simulink model "Mutriku_TD_V5_Data"  (R2017a)
settings: Solver=ode1  StartTime=Times.Ts  StopTime=Times.Tsim  FixedStep=Times.Ts  RelTol=1e-3  EnableMultiTasking=on
values from neighbouring files (symbols this model uses):
  CL = 1    [Plot_Main_Biradiale.m]
undefined symbols (not defined in the file or in its folder): L, Times, Turb, WaveData, WEC
libraries: simulink x1
settings Model: Creator=FixnBock  LastModifiedBy=Temo
settings SolverCC: AlgebraicLoopSolver=LineSearch
settings DataIOCC: LimitDataPoints=on  SaveFormat=StructureWithTime
settings OptimizationCC: DefaultParameterBehavior=Inlined  LifeSpan=inf
settings DebuggingCC: AlgebraicLoopMsg=error  SFUnexpectedBacktrackingDiag=warning  SFNoUnconditionalDefaultTransitionDiag=warning  SFExecutionAtInitializationDiag=none
settings HardwareCC: ProdBitPerSizeT=32  ProdBitPerPtrDiffT=32  ProdWordSize=32  ProdHWDeviceType=Specified
settings ModelReferenceCC: PropagateSignalLabelsOutOfModel=off
settings RTWCC: TemplateMakefile=RTW.MSVCBuild  Description=Create Visual C/C++ Solution File for Simulink Coder
settings GRTTargetCC: TargetLangStandard=C89/C90 (ANSI)
settings ConfigComp: CovMetricSettings=dw  CovHtmlReporting=on  CovSaveCumulativeToWorkspaceVar=on  CovSaveSingleToWorkspaceVar=on  CovExternalEMLEnable=off

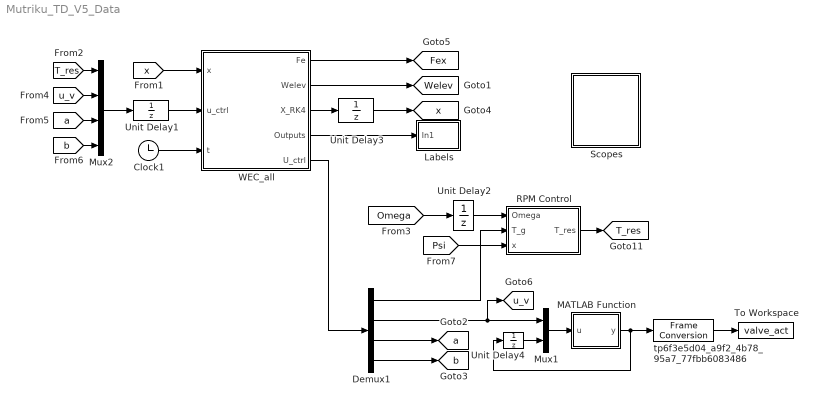
== system Mutriku_TD_V5_Data ==
  Clock1 : Clock
  Demux1 : Demux
  Labels : Subsystem
  MATLAB Function : MATLAB Function  TreatAsAtomicUnit=on
  Mux1 : Mux  Inputs=2
  Mux2 : Mux
  RPM Control : Subsystem
  Scopes : Subsystem
  To Workspace : ToWorkspace  VariableName=valve_act  SampleTime=-1
  Unit Delay1 : UnitDelay  InitialCondition=[0,1,Turb.a,Turb.b]  SampleTime=-1
  Unit Delay2 : UnitDelay  InitialCondition=WEC.Omega0  SampleTime=-1
  Unit Delay3 : UnitDelay  InitialCondition=WEC.X0  SampleTime=-1
  Unit Delay4 : UnitDelay  SampleTime=-1
  WEC_all : MATLAB Function  TreatAsAtomicUnit=on
  tp6f3e5d04_a9f2_4b78_95a7_77fbb6083486 : FrameConversion  InheritSamplingMode=off  OutFrame=Sample-based
  tag scope: Fex=global, T_res=global, Welev=global, a=global, b=global, u_v=global, x=global
  wires:
  tp6f3e5d04_a9f2_4b78_95a7_77fbb6083486/1 -> To Workspace/1
  Unit Delay4/1 -> Mux1/2
  MATLAB Function/1(y) -> Unit Delay4/1, tp6f3e5d04_a9f2_4b78_95a7_77fbb6083486/1
  Mux1/1 -> MATLAB Function/1(u)
  Demux1/2 -> [u_v], Mux1/1
  Demux1/1 -> RPM Control/2(T_g)
  WEC_all/5(U_ctrl) -> Demux1/1
  Clock1/1 -> WEC_all/3(t)
  Unit Delay3/1 -> [x]
  [x] -> WEC_all/1(x)
  WEC_all/4(Outputs) -> Labels/1(In1)
  WEC_all/3(X_RK4) -> Unit Delay3/1
  WEC_all/1(Fe) -> [Fex]
  WEC_all/2(Welev) -> [Welev]
  Demux1/3 -> [a]
  Demux1/4 -> [b]
  [Omega] -> Unit Delay2/1
  Unit Delay2/1 -> RPM Control/1(Omega)
  Mux2/1 -> Unit Delay1/1
  [T_res] -> Mux2/1
  [u_v] -> Mux2/2
  [a] -> Mux2/3
  [b] -> Mux2/4
  Unit Delay1/1 -> WEC_all/2(u_ctrl)
  RPM Control/1(T_res) -> [T_res]
  [Psi] -> RPM Control/3(x)

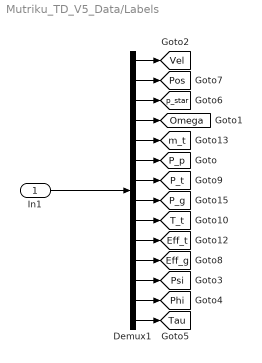
== system Mutriku_TD_V5_Data/Labels ==
  In1 : Inport
  Demux1 : Demux  Outputs=14
  tag scope: Eff_g=global, Eff_t=global, Omega=global, P_g=global, P_p=global, P_t=global, Phi=global, Pos=global, Psi=global, T_t=global, Tau=global, Vel=global, m_t=global, p_star=global
  wires:
  Demux1/5 -> [m_t]
  Demux1/3 -> [p_star]
  Demux1/8 -> [P_g]
  Demux1/1 -> [Vel]
  Demux1/4 -> [Omega]
  Demux1/2 -> [Pos]
  Demux1/9 -> [T_t]
  Demux1/7 -> [P_t]
  Demux1/10 -> [Eff_t]
  Demux1/11 -> [Eff_g]
  Demux1/12 -> [Psi]
  Demux1/13 -> [Phi]
  Demux1/14 -> [Tau]
  Demux1/6 -> [P_p]
  In1/1 -> Demux1/1

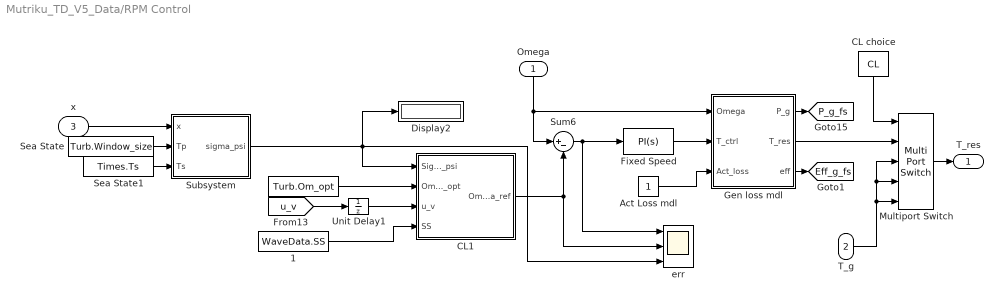
== system Mutriku_TD_V5_Data/RPM Control ==
  Omega : Inport
  T_g : Inport  Port=2
  x : Inport  Port=3
  "    " : Constant  Value=Turb.Om_opt
  "    1" : Constant  Value=WaveData.SS
  Act Loss mdl : Constant
  CL choice : Constant  Value=CL
  CL1 : MATLAB Function  TreatAsAtomicUnit=on
  Display2 : Display
  Fixed Speed : simulink/Continuous/PID Controller  Controller=PI  TimeDomain=Continuous-time  SampleTime=-1  IntegratorMethod=Forward Euler  FilterMethod=Forward Euler  Form=Parallel  UseFilter=on  ControllerParametersSource=internal  P=50  I=0.01  D=0.01  N=100  InitialConditionSource=internal  InitialConditionForIntegrator=0.0  InitialConditionForFilter=0  ExternalReset=none  IgnoreLimit=on  LimitOutput=on  UpperSaturationLimit=Turb.Tmax  LowerSaturationLimit=0  LinearizeAsGain=on  AntiWindupMode=none  Kb=1  TrackingMode=off  Kt=1  PParamMin=[]  PParamMax=[]  IParamMin=[]  IParamMax=[]  DParamMin=[]  DParamMax=[]  NParamMin=[]  NParamMax=[]  KbParamMin=[]  KbParamMax=[]  KtParamMin=[]  KtParamMax=[]  POutMin=[]  POutMax=[]  IOutMin=[]  IOutMax=[]  DOutMin=[]  DOutMax=[]  NOutMin=[]  NOutMax=[]  KbOutMin=[]  KbOutMax=[]  KtOutMin=[]  KtOutMax=[]  IntegratorOutMin=[]  IntegratorOutMax=[]  FilterOutMin=[]  FilterOutMax=[]  SumOutMin=[]  SumOutMax=[]  SumI1OutMin=[]  SumI1OutMax=[]  SumI2OutMin=[]  SumI2OutMax=[]  SumI3OutMin=[]  SumI3OutMax=[]  SumDOutMin=[]  SumDOutMax=[]  SaturationOutMin=[]  SaturationOutMax=[]  IntegratorContinuousStateAttributes=''  IntegratorStateMustResolveToSignalObject=off  IntegratorRTWStateStorageClass=Auto  FilterContinuousStateAttributes=''  FilterStateMustResolveToSignalObject=off  FilterRTWStateStorageClass=Auto  DifferentiatorICPrevScaledInput=0  DifferentiatorOutMin=[]  DifferentiatorOutMax=[]  InitialConditionSetting=State (most efficient)
  Gen loss mdl : MATLAB Function  TreatAsAtomicUnit=on
  Multiport Switch : MultiPortSwitch  Inputs=4  DiagnosticForDefault=None
  Sea State : Constant  Value=Turb.Window_size
  Sea State1 : Constant  Value=Times.Ts
  Subsystem : Subsystem
  Sum6 : Sum  Inputs=|+-
  Unit Delay1 : UnitDelay  InitialCondition=1  SampleTime=-1
  err : Scope  NumInputPorts=3
  T_res : Outport
  tag scope: Eff_g_fs=global, P_g_fs=global
  wires:
  Multiport Switch/1 -> T_res/1
  Omega/1 -> Sum6/1, Gen loss mdl/1(Omega)
  CL choice/1 -> Multiport Switch/1
  CL1/1(Omega_ref) -> Sum6/2, err/2
  T_g/1 -> Multiport Switch/5, Multiport Switch/4, Multiport Switch/3
  Sum6/1 -> Fixed Speed/1, err/1
  Act Loss mdl/1 -> Gen loss mdl/3(Act_loss)
  Gen loss mdl/2(T_res) -> Multiport Switch/2
  Gen loss mdl/1(P_g) -> [P_g_fs]
  Gen loss mdl/3(eff) -> [Eff_g_fs]
  Fixed Speed/1 -> Gen loss mdl/2(T_ctrl)
  "    "/1 -> CL1/2(Omega_opt)
  [u_v] -> Unit Delay1/1
  Unit Delay1/1 -> CL1/3(u_v)
  Sea State/1 -> Subsystem/2(Tp)
  Sea State1/1 -> Subsystem/3(Ts)
  Subsystem/1(sigma_psi) -> err/3, CL1/1(Sigma_psi), Display2/1
  x/1 -> Subsystem/1(x)
  "    1"/1 -> CL1/4(SS)

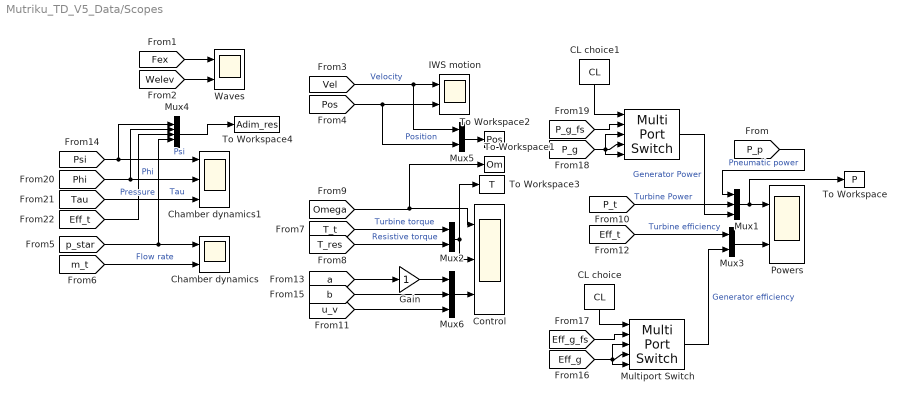
== system Mutriku_TD_V5_Data/Scopes ==
  "    " : MultiPortSwitch  Inputs=4  DiagnosticForDefault=None
  CL choice : Constant  Value=CL
  CL choice1 : Constant  Value=CL
  Chamber dynamics : Scope  NumInputPorts=2
  Chamber dynamics1 : Scope  NumInputPorts=3
  Control : Scope  NumInputPorts=3
  Gain : Gain
  IWS motion : Scope  NumInputPorts=2
  Multiport Switch : MultiPortSwitch  Inputs=4  DiagnosticForDefault=None
  Mux1 : Mux  Inputs=3
  Mux2 : Mux  Inputs=2
  Mux3 : Mux  Inputs=2
  Mux4 : Mux
  Mux5 : Mux  Inputs=2
  Mux6 : Mux  Inputs=3
  Powers : Scope  NumInputPorts=2
  To Workspace : ToWorkspace  VariableName=P  SampleTime=-1
      settings: Decimation=2
  To Workspace1 : ToWorkspace  VariableName=Om  SampleTime=-1
      settings: Decimation=2
  To Workspace2 : ToWorkspace  VariableName=Pos  SampleTime=-1
      settings: Decimation=2
  To Workspace3 : ToWorkspace  VariableName=T  SampleTime=-1
      settings: Decimation=2
  To Workspace4 : ToWorkspace  VariableName=Adim_res  SampleTime=-1
      settings: Decimation=2
  Waves : Scope  NumInputPorts=2
  wires:
  [p_star] -> Mux4/4, Chamber dynamics/1  "Pressure"
  [m_t] -> Chamber dynamics/2  "Flow rate"
  [T_res] -> Mux2/2  "Resistive torque"
  [T_t] -> Mux2/1  "Turbine torque"
  Mux2/1 -> To Workspace3/1, Control/2
  "    "/1 -> Mux1/3  "Generator Power"
  [P_t] -> Mux1/2  "Turbine Power"
  [Eff_t] -> Mux3/1  "Turbine efficiency"
  Mux3/1 -> Powers/2
  Multiport Switch/1 -> Mux3/2  "Generator efficiency"
  Mux1/1 -> To Workspace/1, Powers/1
  [Omega] -> To Workspace1/1, Control/1
  [P_p] -> Mux1/1  "Pneumatic power"
  [Welev] -> Waves/2
  [Fex] -> Waves/1
  Mux6/1 -> Control/3
  [a] -> Gain/1
  [b] -> Mux6/2
  Gain/1 -> Mux6/1
  CL choice/1 -> Multiport Switch/1
  [Eff_g] -> Multiport Switch/5, Multiport Switch/3, Multiport Switch/4
  [Eff_g_fs] -> Multiport Switch/2
  CL choice1/1 -> "    "/1
  [P_g] -> "    "/5, "    "/3, "    "/4
  [P_g_fs] -> "    "/2
  [u_v] -> Mux6/3
  [Psi] -> Mux4/1, Chamber dynamics1/1  "Psi"
  [Tau] -> Chamber dynamics1/3  "Tau"
  Mux4/1 -> To Workspace4/1
  [Eff_t] -> Mux4/3
  [Phi] -> Mux4/2, Chamber dynamics1/2  "Phi"
  [Vel] -> Mux5/1, IWS motion/1  "Velocity"
  [Pos] -> Mux5/2, IWS motion/2  "Position"
  Mux5/1 -> To Workspace2/1

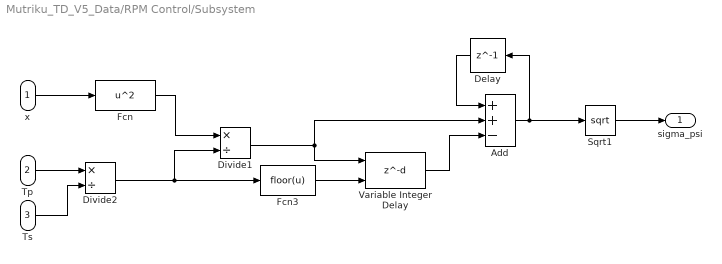
== system Mutriku_TD_V5_Data/RPM Control/Subsystem ==
  x : Inport
  Tp : Inport  Port=2
  Ts : Inport  Port=3
  Add : Sum  Inputs=++-
  Delay : Delay  DelayLength=1  InitialCondition=0
  Divide1 : Product  Inputs=*/
  Divide2 : Product  Inputs=*/
  Fcn : Fcn  Expr=u^2
  Fcn3 : Fcn  Expr=floor(u)
  Sqrt1 : Sqrt  SaturateOnIntegerOverflow=on
  Variable Integer Delay : Delay  DelayLengthSource=Input port  DelayLength=L  DelayLengthUpperLimit=500
      settings: InputPortMap=u0,p1
  sigma_psi : Outport
  wires:
  Divide2/1 -> Divide1/2, Fcn3/1
  Ts/1 -> Divide2/2
  Tp/1 -> Divide2/1
  Fcn/1 -> Divide1/1
  x/1 -> Fcn/1
  Sqrt1/1 -> sigma_psi/1
  Variable Integer Delay/1 -> Add/3
  Divide1/1 -> Add/2, Variable Integer Delay/1
  Delay/1 -> Add/1
  Add/1 -> Sqrt1/1, Delay/1
  Fcn3/1 -> Variable Integer Delay/2

== matlab function Mutriku_TD_V5_Data/WEC_all ==
  data: x input size=24; u_ctrl input size=4; t input; Fe output; WaveData parameter; WEC parameter; Turb parameter; Times parameter; CL parameter; Welev output; X_RK4 output; Outputs output; U_ctrl output size=4
function [Fe,Welev,X_RK4,Outputs, U_ctrl] = main(x,u_ctrl,t,WaveData,WEC,Turb,Times,CL)

Ts = Times.Ts;

[Fexc,Welev] = resource(t,WaveData,WEC,Ts);
Fe = Fexc(3);

[X_RK4,Outputs, U_ctrl] = fcn_rk4(x,Fexc,u_ctrl,WEC,Turb,Ts,CL);

end

function [Fe,welev] = resource(t,WaveData,WEC,Ts)
% Excitation force
smoother = min( 1.0 /  30 * t, 1.0 );
Fe_1  = smoother * WaveData.Wam .* WEC.Fint(1,:) * cos(WaveData.w_discr * (t+Ts) + WEC.Fint(2,:) + WaveData.Wpha)';    
Fe_k  = smoother * WaveData.Wam .* WEC.Fint(1,:) * cos(WaveData.w_discr * (t)    + WEC.Fint(2,:) + WaveData.Wpha)';    
Fe_05 = 0.5 * (Fe_1 + Fe_k);
% Wave elevation
welev = sum(WaveData.Wam * cos(WaveData.w_discr * t + WaveData.Wpha)');
 
Fe = [Fe_1, Fe_05, Fe_k];
end 

function [X_RK4,Outputs, U_ctrl] = fcn_rk4(x,u,u_ctrl,WEC,Turb,Ts,CL)

Fexc_1  = u(1);
Fexc_05 = u(2);
Fexc_k  = u(3);

k1 = fcn_int(x,Fexc_k,u_ctrl, WEC, Turb,CL)*Ts;
k2 = fcn_int(x+k1/2,Fexc_05,u_ctrl, WEC, Turb,CL)*Ts;
k3 = fcn_int(x+k2/2,Fexc_05,u_ctrl, WEC, Turb,CL)*Ts;
k4 = fcn_int(x+k3,Fexc_1,u_ctrl, WEC, Turb,CL)*Ts;

X_RK4 = x + (k1+2*k2+2*k3+k4)/6;

[Outputs, U_ctrl] = fcn_out(X_RK4,u_ctrl,WEC,Turb,CL);
end

function x_dot  = fcn_int(x,u,u_ctrl,WEC,Turb,CL)

% Keeps real part of the state vector and imaginary for the radiation terms
x(1)=real(x(1));
x(2)=real(x(2));
x(3)=real(x(3));
x(4)=real(x(4));

% Get derivate form
x_dot =  WEC.A * x +  WEC.B * u;

% From the state vector
p_star = x(3);
Omega  = x(4);       

% Control
T_ctrl = u_ctrl(1);
u_v = u_ctrl(2);

% Turbine characteristics
Intg_fun = 1;
[P_p, P_t, T_t, Eff_t,m_t] = PTO_Turbine(p_star,Omega,u_v,Intg_fun,WEC,Turb,CL);
% Generator characteristics
Loss_gen = 1;
[P_g, T_res, Eff_g] = PTO_Generator(T_ctrl,Omega,Loss_gen,Turb);

% Volume variation
V   = ( WEC.h_ch - x(2)) *  WEC.S_iws;
dV  = - x(1) *  WEC.S_iws;

%Polytropic 
Kappa = 1/(1-(WEC.beta*Eff_t));
Beta = (Kappa-1)/Kappa;

% p*_dot
% x_dot(3) = - m_t *  WEC.c_at2 / (  WEC.p_at * V )*( p_star + 1.0 )^ WEC.GM1_G ...
%          -  WEC.gamma * ( p_star + 1.0 ) * dV / V;
x_dot(3)= (-Kappa *(p_star+1)*(dV/V)) ...
        - ((Kappa*(p_star+1)^(Beta))*(m_t/(WEC.rho_at*V))) ; 
% Omega_dot
x_dot(4) = (T_t - T_res) / Turb.I; 

% Batch BeP
if CL == 0, x_dot(4) = 0; end

end

function [Sys_out, U_ctrl] = fcn_out(x,u_ctrl,WEC,Turb,CL)

% Initialise output vector size
Sys_out = zeros(14,1);
% U_ctrl  = zeros(4,1); 

% From the state vector
vel   = real(x(1));
pos   = real(x(2));
p_star= real(x(3));
Omega  = real(x(4));

if CL
    % Control vector
    if Omega > Turb.Om_Tci
        T_ctrl = u_ctrl(3) * Omega ^u_ctrl(4);
    else
        T_ctrl = 0;
    end
    u_v = u_ctrl(2);

    % Turbine characteristics
    Intg_fun = 0;
    [P_p, P_t, T_t, Eff_t,m_t,valve_pos,Psi,Phi,Tau] = PTO_Turbine(p_star,Omega,u_v,Intg_fun,WEC,Turb,CL);
    % Generator characteristics
    Loss_gen = 1;
    [P_g, T_res, Eff_g] = PTO_Generator(T_ctrl,Omega,Loss_gen,Turb);
else 
    Omega = Turb.Om_opt;    
    u_v = u_ctrl(2);
    Intg_fun = 0;
    [P_p, P_t, T_t, Eff_t,m_t,valve_pos,Psi,Phi,Tau] = PTO_Turbine(p_star,Omega,u_v,Intg_fun,WEC,Turb,0);
    P_g = 0; T_res = 0; Eff_g = 0;
end

% Outputs
Sys_out(1) = vel;
Sys_out(2) = pos;
Sys_out(3) = p_star;
Sys_out(4) = Omega;
Sys_out(5) = m_t;
Sys_out(6) = P_p;
Sys_out(7) = P_t;
Sys_out(8) = P_g;
Sys_out(9) = T_t;
Sys_out(10) = Eff_t; 
Sys_out(11) = Eff_g;
Sys_out(12) = Psi; 
Sys_out(13) = Phi;
Sys_out(14) = Tau;

U_ctrl = [T_res; valve_pos; u_ctrl(3); u_ctrl(4)];
end

== matlab function Mutriku_TD_V5_Data/RPM Control/Gen loss mdl ==
  data: Omega input; T_ctrl input; P_g output; Act_loss input; Turb parameter; T_res output; eff output
function [P_g, T_res, eff] = PTO_Generator(Omega,T_ctrl,Act_loss,Turb)

Omega_thr = Turb.over_speed * Turb.Om_nom;
    
% Generator operation ranges
if (Omega > 0.1*Turb.Om_nom) && (Omega <= Omega_thr)
    if T_ctrl > Turb.Tmax
        T_e = Turb.Tmax; 
    else T_e = T_ctrl;
    end
% Extremum operation range Om < Om_min and Om > Om_max    
elseif  Omega <= 0.05*Turb.Om_nom || Omega > Turb.Om_max
    T_e = Turb.Mech_loss/Omega;
% Flux-weakening region, or loss of capacity of peak electrical torque
else
    tmax_os = Turb.Tmax * (Omega_thr / Omega)^2;
    if T_ctrl > tmax_os
        T_e = tmax_os;
    else T_e = T_ctrl;
    end
end

% Actualise Power
P_out =  T_e*Omega;

% From Obeki curves, Endika
cosphi = 8e-15*P_out^3 - 1e-9*P_out^2 + 5e-5*P_out + 0.087;
if cosphi > 1, cosphi = 1; end

% Actualise instaneaous voltage
if Omega < Omega_thr
    f_hz =(Turb.nb_pp * Omega * 30/pi)/60;
    v_act = Turb.Vslope * f_hz; 
else
    f_hz = Turb.F_hz;
    v_act = Turb.Vmax;
end

I_l = P_out / (sqrt(3)*cosphi*v_act); 

%% Losses calculation
if Act_loss == 1
        Wind_loss = I_l^2 * Turb.R_ohm;    % Windings losses
        Fe_loss = Turb.Flux_dens^2 * ...
            (Turb.Kh*f_hz/100 + ...
             Turb.Kk*(Turb.Thick_max*f_hz/100)^2) * 0.6 * Turb.Weight; 
        % (W) Losses in Hysteresis & Foucault, assuming iron core 50% of the weight
        P_loss = Turb.Mech_loss + Wind_loss + Fe_loss;       
        eff = 1 - P_loss/P_out;
                
        T_loss = P_loss / Omega;

        P_g = eff * sqrt(3) * v_act * I_l * cosphi;

    if eff < 0 
        P_loss = Turb.Mech_loss;
        P_g = 0;
        eff = 0.0;        
        T_loss = P_loss / Omega; 
    end
    
else
    T_loss = 0;
    eff = 1.0; 
    P_g = P_out;
end

%if Turb.Turb == 1 && Omega <= 40, T_e = 0; end

T_res = T_e + T_loss;

end

== matlab function Mutriku_TD_V5_Data/RPM Control/CL1 ==
  data: Sigma_psi input; Omega_opt input; u_v input; Omega_ref output; Turb parameter; SS input
function Omega_ref = fcn(Sigma_psi,Omega_opt,u_v,Turb,SS)
SigPsi_tab = 1.25*[866 969 1154 1453 1686 2081 2498 2853 3284 3699 4244 4354 4394 4444]; % 1.25* 17.29
if u_v == 1
    Omega_ref = Omega_opt;
    Omega_ref = Sigma_psi * Turb.k_sigpsi ; %SigPsi_tab(SS);% 1.5*k_sigpsi => 17.78
else 
    Omega_ref = Turb.Om_ci*0.95;
end

== matlab function Mutriku_TD_V5_Data/MATLAB Function ==
  data: u input size=2; y output size=1
function y = fcn(u)
%#codegen
if u(1) == 0
    y = u(2) + 1;
else y = u(2);
end
